simulink model "UZ_D_GaN_Inverter_reduced"  (R2020b)
settings: Solver=FixedStepDiscrete  StartTime=0.0  StopTime=300e-6  RelTol=1e-3
libraries: simulink x8, hdlsllib x2
settings Model: DataTypeOverride=Off  Creator=Michael Hoerner  LastModifiedBy=Michael Hoerner
settings DataIOCC: LimitDataPoints=on  SaveOutput=off  SaveTime=off
settings OptimizationCC: BlockReduction=off  ConditionallyExecuteInputs=off  DefaultParameterBehavior=Inlined  LifeSpan=inf
settings DebuggingCC: AlgebraicLoopMsg=error  SingleTaskRateTransMsg=error  AllowSymbolicDim=off  StrictBusMsg=ErrorOnBusTreatedAsVector  SFUnexpectedBacktrackingDiag=warning  SFNoUnconditionalDefaultTransitionDiag=warning  SFExecutionAtInitializationDiag=none  ArithmeticOperatorsInVariantConditions=warning
settings HardwareCC: ProdBitPerPointer=32  ProdBitPerSizeT=32  ProdBitPerPtrDiffT=32  ProdLargestAtomicFloat=None  ProdIntDivRoundTo=Undefined  ProdEndianess=Unspecified  ProdWordSize=32  ProdHWDeviceType=ASIC/FPGA->ASIC/FPGA  ProdEqTarget=off
settings SFSimCC: SimUseLocalCustomCode=off  CustomCodeUndefinedFunction=UseInterfaceOnly
settings RTWCC: RTWUseLocalCustomCode=off
settings CodeAppCC: StateflowObjectComments=on
settings GRTTargetCC: TargetLangStandard=C89/C90 (ANSI)
settings ConfigComp: CovScope=ReferencedModels  CovMetricSettings=dw  CovSaveCumulativeToWorkspaceVar=on  CovSaveSingleToWorkspaceVar=on  CovExternalEMLEnable=off  CovSFcnEnable=off

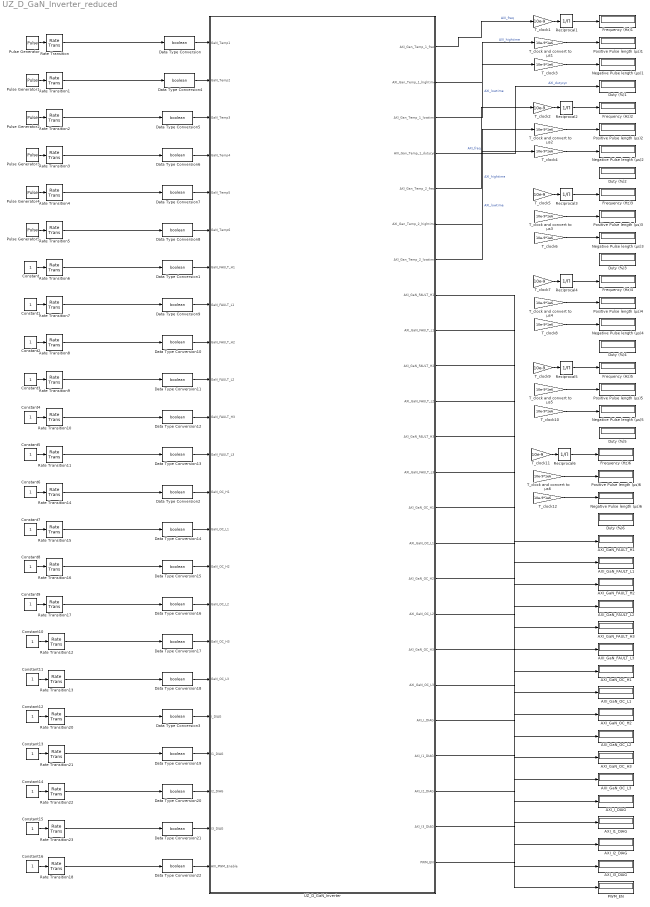
== system UZ_D_GaN_Inverter_reduced ==
  AXI_GaN_FAULT_H1 : Display
  AXI_GaN_FAULT_H2 : Display
  AXI_GaN_FAULT_H3 : Display
  AXI_GaN_FAULT_L1 : Display
  AXI_GaN_FAULT_L2 : Display
  AXI_GaN_FAULT_L3 : Display
  AXI_GaN_OC_H1 : Display
  AXI_GaN_OC_H2 : Display
  AXI_GaN_OC_H3 : Display
  AXI_GaN_OC_L1 : Display
  AXI_GaN_OC_L2 : Display
  AXI_GaN_OC_L3 : Display
  AXI_I1_DIAG : Display
  AXI_I2_DIAG : Display
  AXI_I3_DIAG : Display
  AXI_I_DIAG : Display
  Constant{,1..16} (17 alike) : Constant
  Data Type Conversion{,1..22} (23 alike) : DataTypeConversion  OutDataTypeStr=boolean
  Duty (%){1..6} (6 alike) : Display
  Frequency (Hz){1..6} (6 alike) : Display
  Negative Pulse length (µs){1..6} (6 alike) : Display
  PWM_EN : Display
  Positive Pulse length (µs){1..6} (6 alike) : Display
  Pulse Generator : DiscretePulseGenerator  PulseType=Time based  Period=1/10000  PulseWidth=7
  Pulse Generator1 : DiscretePulseGenerator  PulseType=Time based  Period=1/10000  PulseWidth=8
  Pulse Generator2 : DiscretePulseGenerator  PulseType=Time based  Period=1/10000  PulseWidth=9
  Pulse Generator3 : DiscretePulseGenerator  PulseType=Time based  Period=1/10000  PulseWidth=10
  Pulse Generator4 : DiscretePulseGenerator  PulseType=Time based  Period=1/10000  PulseWidth=11
  Pulse Generator5 : DiscretePulseGenerator  PulseType=Time based  Period=1/10000  PulseWidth=12
  Rate Transition{,1..18,20..23} (23 alike) : RateTransition  OutPortSampleTime=10e-9
  Reciprocal{1..6} (6 alike) : Product  Inputs=/
  T_clock and convert to µs{1..6} (6 alike) : Gain  Gain=10e-9*1e6
  T_clock{1..2,5,7,9,11} (6 alike) : Gain  Gain=10e-9
  T_clock{3..4,6,8,10,12} (6 alike) : Gain  Gain=10e-9*1e6
  UZ_D_GaN_Inverter : Subsystem  TreatAsAtomicUnit=on
  wires:
  Data Type Conversion/1 -> UZ_D_GaN_Inverter/1(GaN_Temp1)
  Pulse Generator/1 -> Rate Transition/1
  Pulse Generator1/1 -> Rate Transition1/1
  Pulse Generator2/1 -> Rate Transition2/1
  Pulse Generator3/1 -> Rate Transition3/1
  Pulse Generator4/1 -> Rate Transition4/1
  Pulse Generator5/1 -> Rate Transition5/1
  Rate Transition/1 -> Data Type Conversion/1
  Rate Transition1/1 -> Data Type Conversion4/1
  Rate Transition2/1 -> Data Type Conversion5/1
  Rate Transition3/1 -> Data Type Conversion6/1
  Rate Transition4/1 -> Data Type Conversion7/1
  Rate Transition5/1 -> Data Type Conversion8/1
  Rate Transition9/1 -> Data Type Conversion11/1
  Rate Transition11/1 -> Data Type Conversion13/1
  Rate Transition6/1 -> Data Type Conversion1/1
  Rate Transition10/1 -> Data Type Conversion12/1
  Rate Transition8/1 -> Data Type Conversion10/1
  Rate Transition7/1 -> Data Type Conversion9/1
  Data Type Conversion1/1 -> UZ_D_GaN_Inverter/7(GaN_FAULT_H1)
  Rate Transition12/1 -> Data Type Conversion17/1
  Rate Transition14/1 -> Data Type Conversion2/1
  Rate Transition15/1 -> Data Type Conversion14/1
  Rate Transition17/1 -> Data Type Conversion16/1
  Data Type Conversion2/1 -> UZ_D_GaN_Inverter/13(GaN_OC_H1)
  Rate Transition13/1 -> Data Type Conversion18/1
  Rate Transition16/1 -> Data Type Conversion15/1
  Rate Transition20/1 -> Data Type Conversion3/1
  Rate Transition21/1 -> Data Type Conversion19/1
  Rate Transition23/1 -> Data Type Conversion21/1
  Data Type Conversion3/1 -> UZ_D_GaN_Inverter/19(I_DIAG)
  Rate Transition22/1 -> Data Type Conversion20/1
  Constant/1 -> Rate Transition6/1
  Constant1/1 -> Rate Transition7/1
  Constant2/1 -> Rate Transition8/1
  Constant3/1 -> Rate Transition9/1
  Constant4/1 -> Rate Transition10/1
  Constant5/1 -> Rate Transition11/1
  Constant9/1 -> Rate Transition17/1
  Constant7/1 -> Rate Transition15/1
  Constant10/1 -> Rate Transition12/1
  Constant8/1 -> Rate Transition16/1
  Constant11/1 -> Rate Transition13/1
  Constant6/1 -> Rate Transition14/1
  Constant15/1 -> Rate Transition23/1
  Constant13/1 -> Rate Transition21/1
  Constant14/1 -> Rate Transition22/1
  Constant12/1 -> Rate Transition20/1
  T_clock and convert to µs1/1 -> Positive Pulse length (µs)1/1
  T_clock3/1 -> Negative Pulse length (µs)1/1
  Reciprocal1/1 -> Frequency (Hz)1/1
  UZ_D_GaN_Inverter/3(AXI_Gan_Temp_1_lowtime) -> T_clock3/1  "AXI_lowtime"
  UZ_D_GaN_Inverter/2(AXI_Gan_Temp_1_hightime) -> T_clock and convert to µs1/1  "AXI_hightime"
  T_clock1/1 -> Reciprocal1/1
  UZ_D_GaN_Inverter/1(AXI_Gan_Temp_1_freq) -> T_clock1/1  "AXI_freq"
  UZ_D_GaN_Inverter/4(AXI_Gan_Temp_1_dutycyc) -> Duty (%)1/1  "AXI_dutycyc"
  UZ_D_GaN_Inverter/7(AXI_Gan_Temp_2_lowtime) -> T_clock4/1  "AXI_lowtime"
  T_clock2/1 -> Reciprocal2/1
  ? -> Duty (%)2/1  "AXI_dutycyc"
  Reciprocal2/1 -> Frequency (Hz)2/1
  T_clock4/1 -> Negative Pulse length (µs)2/1
  UZ_D_GaN_Inverter/6(AXI_Gan_Temp_2_hightime) -> T_clock and convert to µs2/1  "AXI_hightime"
  T_clock and convert to µs2/1 -> Positive Pulse length (µs)2/1
  UZ_D_GaN_Inverter/5(AXI_Gan_Temp_2_freq) -> T_clock2/1  "AXI_freq"
  ? -> T_clock6/1  "AXI_lowtime"
  T_clock5/1 -> Reciprocal3/1
  ? -> Duty (%)3/1  "AXI_dutycyc"
  Reciprocal3/1 -> Frequency (Hz)3/1
  T_clock6/1 -> Negative Pulse length (µs)3/1
  ? -> T_clock and convert to µs3/1  "AXI_hightime"
  T_clock and convert to µs3/1 -> Positive Pulse length (µs)3/1
  ? -> T_clock5/1  "AXI_freq"
  ? -> T_clock8/1  "AXI_lowtime"
  T_clock7/1 -> Reciprocal4/1
  ? -> Duty (%)4/1  "AXI_dutycyc"
  Reciprocal4/1 -> Frequency (Hz)4/1
  T_clock8/1 -> Negative Pulse length (µs)4/1
  ? -> T_clock and convert to µs4/1  "AXI_hightime"
  T_clock and convert to µs4/1 -> Positive Pulse length (µs)4/1
  ? -> T_clock7/1  "AXI_freq"
  ? -> T_clock10/1  "AXI_lowtime"
  T_clock9/1 -> Reciprocal5/1
  ? -> Duty (%)5/1  "AXI_dutycyc"
  Reciprocal5/1 -> Frequency (Hz)5/1
  T_clock10/1 -> Negative Pulse length (µs)5/1
  ? -> T_clock and convert to µs5/1  "AXI_hightime"
  T_clock and convert to µs5/1 -> Positive Pulse length (µs)5/1
  ? -> T_clock9/1  "AXI_freq"
  ? -> T_clock12/1  "AXI_lowtime"
  T_clock11/1 -> Reciprocal6/1
  ? -> Duty (%)6/1  "AXI_dutycyc"
  Reciprocal6/1 -> Frequency (Hz)6/1
  T_clock12/1 -> Negative Pulse length (µs)6/1
  ? -> T_clock and convert to µs6/1  "AXI_hightime"
  T_clock and convert to µs6/1 -> Positive Pulse length (µs)6/1
  ? -> T_clock11/1  "AXI_freq"
  UZ_D_GaN_Inverter/8(AXI_GaN_FAULT_H1) -> AXI_GaN_FAULT_H1/1
  UZ_D_GaN_Inverter/9(AXI_GaN_FAULT_L1) -> AXI_GaN_FAULT_L1/1
  UZ_D_GaN_Inverter/10(AXI_GaN_FAULT_H2) -> AXI_GaN_FAULT_H2/1
  UZ_D_GaN_Inverter/11(AXI_GaN_FAULT_L2) -> AXI_GaN_FAULT_L2/1
  UZ_D_GaN_Inverter/12(AXI_GaN_FAULT_H3) -> AXI_GaN_FAULT_H3/1
  UZ_D_GaN_Inverter/13(AXI_GaN_FAULT_L3) -> AXI_GaN_FAULT_L3/1
  UZ_D_GaN_Inverter/14(AXI_GaN_OC_H1) -> AXI_GaN_OC_H1/1
  UZ_D_GaN_Inverter/15(AXI_GaN_OC_L1) -> AXI_GaN_OC_L1/1
  UZ_D_GaN_Inverter/16(AXI_GaN_OC_H2) -> AXI_GaN_OC_H2/1
  UZ_D_GaN_Inverter/17(AXI_GaN_OC_L2) -> AXI_GaN_OC_L2/1
  UZ_D_GaN_Inverter/18(AXI_GaN_OC_H3) -> AXI_GaN_OC_H3/1
  UZ_D_GaN_Inverter/19(AXI_GaN_OC_L3) -> AXI_GaN_OC_L3/1
  UZ_D_GaN_Inverter/20(AXI_I_DIAG) -> AXI_I_DIAG/1
  UZ_D_GaN_Inverter/21(AXI_I1_DIAG) -> AXI_I1_DIAG/1
  UZ_D_GaN_Inverter/22(AXI_I2_DIAG) -> AXI_I2_DIAG/1
  UZ_D_GaN_Inverter/23(AXI_I3_DIAG) -> AXI_I3_DIAG/1
  Data Type Conversion4/1 -> UZ_D_GaN_Inverter/2(GaN_Temp2)
  Data Type Conversion5/1 -> UZ_D_GaN_Inverter/3(GaN_Temp3)
  Data Type Conversion6/1 -> UZ_D_GaN_Inverter/4(GaN_Temp4)
  Data Type Conversion7/1 -> UZ_D_GaN_Inverter/5(GaN_Temp5)
  Data Type Conversion8/1 -> UZ_D_GaN_Inverter/6(GaN_Temp6)
  Data Type Conversion9/1 -> UZ_D_GaN_Inverter/8(GaN_FAULT_L1)
  Data Type Conversion10/1 -> UZ_D_GaN_Inverter/9(GaN_FAULT_H2)
  Data Type Conversion11/1 -> UZ_D_GaN_Inverter/10(GaN_FAULT_L2)
  Data Type Conversion12/1 -> UZ_D_GaN_Inverter/11(GaN_FAULT_H3)
  Data Type Conversion13/1 -> UZ_D_GaN_Inverter/12(GaN_FAULT_L3)
  Data Type Conversion14/1 -> UZ_D_GaN_Inverter/14(GaN_OC_L1)
  Data Type Conversion15/1 -> UZ_D_GaN_Inverter/15(GaN_OC_H2)
  Data Type Conversion16/1 -> UZ_D_GaN_Inverter/16(GaN_OC_L2)
  Data Type Conversion17/1 -> UZ_D_GaN_Inverter/17(GaN_OC_H3)
  Data Type Conversion18/1 -> UZ_D_GaN_Inverter/18(GaN_OC_L3)
  Data Type Conversion19/1 -> UZ_D_GaN_Inverter/20(I1_DIAG)
  Data Type Conversion20/1 -> UZ_D_GaN_Inverter/21(I2_DIAG)
  Data Type Conversion21/1 -> UZ_D_GaN_Inverter/22(I3_DIAG)
  Data Type Conversion22/1 -> UZ_D_GaN_Inverter/23(AXI_PWM_Enable)
  Constant16/1 -> Rate Transition18/1
  Rate Transition18/1 -> Data Type Conversion22/1
  UZ_D_GaN_Inverter/24(PWM_EN) -> PWM_EN/1

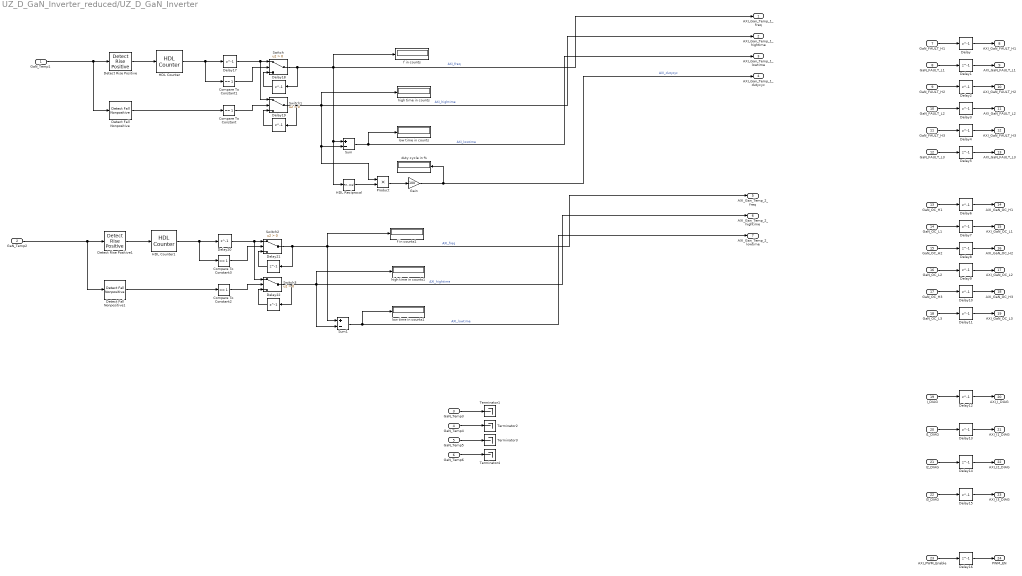
== system UZ_D_GaN_Inverter_reduced/UZ_D_GaN_Inverter ==
  GaN_Temp1 : Inport  OutDataTypeStr=boolean
  GaN_Temp2 : Inport  Port=2  OutDataTypeStr=boolean
  GaN_Temp3 : Inport  Port=3  OutDataTypeStr=boolean
  GaN_Temp4 : Inport  Port=4  OutDataTypeStr=boolean
  GaN_Temp5 : Inport  Port=5  OutDataTypeStr=boolean
  GaN_Temp6 : Inport  Port=6  OutDataTypeStr=boolean
  GaN_FAULT_H1 : Inport  Port=7  OutDataTypeStr=boolean
  GaN_FAULT_L1 : Inport  Port=8  OutDataTypeStr=boolean
  GaN_FAULT_H2 : Inport  Port=9  OutDataTypeStr=boolean
  GaN_FAULT_L2 : Inport  Port=10  OutDataTypeStr=boolean
  GaN_FAULT_H3 : Inport  Port=11  OutDataTypeStr=boolean
  GaN_FAULT_L3 : Inport  Port=12  OutDataTypeStr=boolean
  GaN_OC_H1 : Inport  Port=13  OutDataTypeStr=boolean
  GaN_OC_L1 : Inport  Port=14  OutDataTypeStr=boolean
  GaN_OC_H2 : Inport  Port=15  OutDataTypeStr=boolean
  GaN_OC_L2 : Inport  Port=16  OutDataTypeStr=boolean
  GaN_OC_H3 : Inport  Port=17  OutDataTypeStr=boolean
  GaN_OC_L3 : Inport  Port=18  OutDataTypeStr=boolean
  I_DIAG : Inport  Port=19  OutDataTypeStr=boolean
  I1_DIAG : Inport  Port=20  OutDataTypeStr=boolean
  I2_DIAG : Inport  Port=21  OutDataTypeStr=boolean
  I3_DIAG : Inport  Port=22  OutDataTypeStr=boolean
  AXI_PWM_Enable : Inport  Port=23  OutDataTypeStr=boolean
  Compare To Constant{,1..3} (4 alike) : simulink/Logic and Bit Operations/Compare To Constant  relop===  const=1  OutDataTypeStr=boolean
  Delay{,1..22} (23 alike) : Delay  DelayLength=1
  Detect Fall Nonpositive : simulink/Logic and Bit Operations/Detect Fall Nonpositive  vinit=0  OutDataTypeStr=boolean
      settings: SourceProductBaseCode=SL
  Detect Fall Nonpositive1 : simulink/Logic and Bit Operations/Detect Fall Nonpositive  vinit=0  OutDataTypeStr=boolean
      settings: SourceProductBaseCode=SL
  Detect Rise Positive : simulink/Logic and Bit Operations/Detect Rise Positive  vinit=0  OutDataTypeStr=boolean
  Detect Rise Positive1 : simulink/Logic and Bit Operations/Detect Rise Positive  vinit=0  OutDataTypeStr=boolean
  Gain : Gain  Gain=100  OutDataTypeStr=fixdt(1,32,24)
  HDL Counter : hdlsllib/Sources/HDL Counter  CountType=Count limited  CountInit=1  CountStep=1  CountMax=2500000  CountFromType=Specify  CountFrom=1  CountResetPort=on  CountLoadPort=off  CountEnbPort=off  CountDirPort=off  CountDataType=Unsigned  CountWordLen=32  CountFracLen=0  CountSampTime=1
  HDL Counter1 : hdlsllib/Sources/HDL Counter  CountType=Count limited  CountInit=1  CountStep=1  CountMax=2500000  CountFromType=Specify  CountFrom=1  CountResetPort=on  CountLoadPort=off  CountEnbPort=off  CountDirPort=off  CountDataType=Unsigned  CountWordLen=32  CountFracLen=0  CountSampTime=1
  HDL Reciprocal : Reciprocal
  Product : Product  OutDataTypeStr=fixdt(1,32,30)
  Sum : Sum  Inputs=+-  AccumDataTypeStr=uint32
  Sum1 : Sum  Inputs=+-  AccumDataTypeStr=uint32
  Switch{,1..3} (4 alike) : Switch  Criteria=u2 > Threshold
  Terminator{1..4} (4 alike) : Terminator
  duty cycle in % : Display
  f in counts : Display
  f in counts1 : Display
  high time in counts : Display
  high time in counts1 : Display
  low time in counts : Display
  low time in counts1 : Display
  AXI_Gan_Temp_1_freq : Outport  PortDimensions=1  VectorParamsAs1DForOutWhenUnconnected=off
  AXI_Gan_Temp_1_hightime : Outport  Port=2  PortDimensions=1  VectorParamsAs1DForOutWhenUnconnected=off
  AXI_Gan_Temp_1_lowtime : Outport  Port=3  PortDimensions=1  VectorParamsAs1DForOutWhenUnconnected=off
  AXI_Gan_Temp_1_dutycyc : Outport  Port=4  PortDimensions=1  VectorParamsAs1DForOutWhenUnconnected=off
  AXI_Gan_Temp_2_freq : Outport  Port=5  PortDimensions=1  VectorParamsAs1DForOutWhenUnconnected=off
  AXI_Gan_Temp_2_hightime : Outport  Port=6  PortDimensions=1  VectorParamsAs1DForOutWhenUnconnected=off
  AXI_Gan_Temp_2_lowtime : Outport  Port=7  PortDimensions=1  VectorParamsAs1DForOutWhenUnconnected=off
  AXI_GaN_FAULT_H1 : Outport  Port=8  PortDimensions=1  VectorParamsAs1DForOutWhenUnconnected=off
  AXI_GaN_FAULT_L1 : Outport  Port=9  PortDimensions=1  VectorParamsAs1DForOutWhenUnconnected=off
  AXI_GaN_FAULT_H2 : Outport  Port=10  PortDimensions=1  VectorParamsAs1DForOutWhenUnconnected=off
  AXI_GaN_FAULT_L2 : Outport  Port=11  PortDimensions=1  VectorParamsAs1DForOutWhenUnconnected=off
  AXI_GaN_FAULT_H3 : Outport  Port=12  PortDimensions=1  VectorParamsAs1DForOutWhenUnconnected=off
  AXI_GaN_FAULT_L3 : Outport  Port=13  PortDimensions=1  VectorParamsAs1DForOutWhenUnconnected=off
  AXI_GaN_OC_H1 : Outport  Port=14  PortDimensions=1  VectorParamsAs1DForOutWhenUnconnected=off
  AXI_GaN_OC_L1 : Outport  Port=15  PortDimensions=1  VectorParamsAs1DForOutWhenUnconnected=off
  AXI_GaN_OC_H2 : Outport  Port=16  PortDimensions=1  VectorParamsAs1DForOutWhenUnconnected=off
  AXI_GaN_OC_L2 : Outport  Port=17  PortDimensions=1  VectorParamsAs1DForOutWhenUnconnected=off
  AXI_GaN_OC_H3 : Outport  Port=18  PortDimensions=1  VectorParamsAs1DForOutWhenUnconnected=off
  AXI_GaN_OC_L3 : Outport  Port=19  PortDimensions=1  VectorParamsAs1DForOutWhenUnconnected=off
  AXI_I_DIAG : Outport  Port=20  PortDimensions=1  VectorParamsAs1DForOutWhenUnconnected=off
  AXI_I1_DIAG : Outport  Port=21  PortDimensions=1  VectorParamsAs1DForOutWhenUnconnected=off
  AXI_I2_DIAG : Outport  Port=22  PortDimensions=1  VectorParamsAs1DForOutWhenUnconnected=off
  AXI_I3_DIAG : Outport  Port=23  PortDimensions=1  VectorParamsAs1DForOutWhenUnconnected=off
  PWM_EN : Outport  Port=24  PortDimensions=1  VectorParamsAs1DForOutWhenUnconnected=off
  wires:
  Switch/1 -> AXI_Gan_Temp_1_freq/1, HDL Reciprocal/1, Sum/1, f in counts/1, Delay18/1  "AXI_freq"
  Switch1/1 -> AXI_Gan_Temp_1_hightime/1, Product/1, Sum/2, high time in counts/1, Delay19/1  "AXI_hightime"
  Sum/1 -> AXI_Gan_Temp_1_lowtime/1, low time in counts/1  "AXI_lowtime"
  Gain/1 -> AXI_Gan_Temp_1_dutycyc/1, duty cycle in %/1  "AXI_dutycyc"
  GaN_OC_H1/1 -> Delay6/1
  GaN_OC_L1/1 -> Delay7/1
  GaN_OC_H2/1 -> Delay8/1
  GaN_OC_L2/1 -> Delay9/1
  GaN_OC_H3/1 -> Delay10/1
  GaN_OC_L3/1 -> Delay11/1
  I_DIAG/1 -> Delay12/1
  I1_DIAG/1 -> Delay13/1
  I2_DIAG/1 -> Delay14/1
  I3_DIAG/1 -> Delay15/1
  GaN_FAULT_H1/1 -> Delay/1
  GaN_FAULT_L1/1 -> Delay1/1
  GaN_FAULT_H2/1 -> Delay2/1
  GaN_FAULT_L2/1 -> Delay3/1
  GaN_FAULT_L3/1 -> Delay5/1
  GaN_FAULT_H3/1 -> Delay4/1
  AXI_PWM_Enable/1 -> Delay16/1
  Delay/1 -> AXI_GaN_FAULT_H1/1
  Delay1/1 -> AXI_GaN_FAULT_L1/1
  Delay2/1 -> AXI_GaN_FAULT_H2/1
  Delay3/1 -> AXI_GaN_FAULT_L2/1
  Delay4/1 -> AXI_GaN_FAULT_H3/1
  Delay5/1 -> AXI_GaN_FAULT_L3/1
  Delay6/1 -> AXI_GaN_OC_H1/1
  Delay7/1 -> AXI_GaN_OC_L1/1
  Delay9/1 -> AXI_GaN_OC_L2/1
  Delay8/1 -> AXI_GaN_OC_H2/1
  Delay10/1 -> AXI_GaN_OC_H3/1
  Delay11/1 -> AXI_GaN_OC_L3/1
  Delay12/1 -> AXI_I_DIAG/1
  Delay13/1 -> AXI_I1_DIAG/1
  Delay14/1 -> AXI_I2_DIAG/1
  Delay15/1 -> AXI_I3_DIAG/1
  Delay16/1 -> PWM_EN/1
  Delay19/1 -> Switch1/3
  Detect Rise Positive/1 -> HDL Counter/1
  HDL Reciprocal/1 -> Product/2
  Compare To Constant1/1 -> Switch/2
  GaN_Temp1/1 -> Detect Fall Nonpositive/1, Detect Rise Positive/1
  Compare To Constant/1 -> Switch1/2
  Detect Fall Nonpositive/1 -> Compare To Constant/1
  Delay18/1 -> Switch/3
  Delay17/1 -> Switch1/1, Switch/1
  Product/1 -> Gain/1
  HDL Counter/1 -> Compare To Constant1/1, Delay17/1
  GaN_Temp3/1 -> Terminator1/1
  GaN_Temp4/1 -> Terminator2/1
  GaN_Temp5/1 -> Terminator3/1
  GaN_Temp6/1 -> Terminator4/1
  Compare To Constant2/1 -> Switch3/2
  Delay20/1 -> Switch3/1, Switch2/1
  GaN_Temp2/1 -> Detect Fall Nonpositive1/1, Detect Rise Positive1/1
  Delay22/1 -> Switch3/3
  Compare To Constant3/1 -> Switch2/2
  Detect Rise Positive1/1 -> HDL Counter1/1
  HDL Counter1/1 -> Compare To Constant3/1, Delay20/1
  Switch2/1 -> AXI_Gan_Temp_2_freq/1, Sum1/1, f in counts1/1, Delay21/1  "AXI_freq"
  Sum1/1 -> AXI_Gan_Temp_2_lowtime/1, low time in counts1/1  "AXI_lowtime"
  Delay21/1 -> Switch2/3
  Switch3/1 -> AXI_Gan_Temp_2_hightime/1, Sum1/2, high time in counts1/1, Delay22/1  "AXI_hightime"
  Detect Fall Nonpositive1/1 -> Compare To Constant2/1
